simulink model "bb_pid_hg_sl"  (Simulink 7.9)
settings: Solver=FixedStepDiscrete  StartTime=0.0  StopTime=inf  FixedStep=ts  RelTol=1e-3
values from neighbouring files (symbols this model uses):
  K_theta_hg = (pi/180)*(2.1/15)    (= 0.00244346095279)    [bb_lqr_hg.m]    (also in bb_lqr_servo_hg.m; bb_lqr_test.m; bb_pid_hg.m)
  Kd = -((p1+p2)*T + 1)/K    [bb_pid_hg.m]    (also in sim_param.mat = 0)
  kd = -(p1+p2+p3)/K_b    [bb_pid_hg.m]    (also in bb_pid_rc.m)
  kff = ki/alpha    [bb_pid_hg.m]    (also in bb_pid_rc.m)
  ki = -p1*p2*p3/K_b    [bb_pid_hg.m]    (also in bb_pid_rc.m)
  Kp = p1*p2*T/K    [bb_pid_hg.m]    (also in sim_param.mat = 0)
  kp = (p1*p2 + p2*p3 + p3*p1)/K_b    [bb_pid_hg.m]    (also in bb_pid_rc.m)
  r = 60    [sim_param.mat]
  r1 = 20    [bb_lqr_hg.m]    (also in bb_lqr_servo_hg.m = 15; bb_pid_hg.m = 15; bb_pid_rc.m = 15)
  r2 = 20    [bb_lqr_hg.m]    (also in bb_lqr_servo_hg.m = 25; bb_pid_hg.m = 25; bb_pid_rc.m = 25)
  r_cyc = 4    [sim_param.mat]
  ts = 0.02    [sim_param.mat]
undefined symbols (not defined in the file or in its folder): denbd, denlpf, denpd, DiscIntNeverNeededParam, numbd, numlpf, numpd
libraries: arduino_io_lib x6, simulink x6
settings Model: Creator=hirata  LastModifiedBy=hirata
settings DebuggingCC: FcnCallInpInsideContextMsg=Use local settings
settings GRTTargetCC: CombineOutputUpdateFcns=off  GRTInterface=on

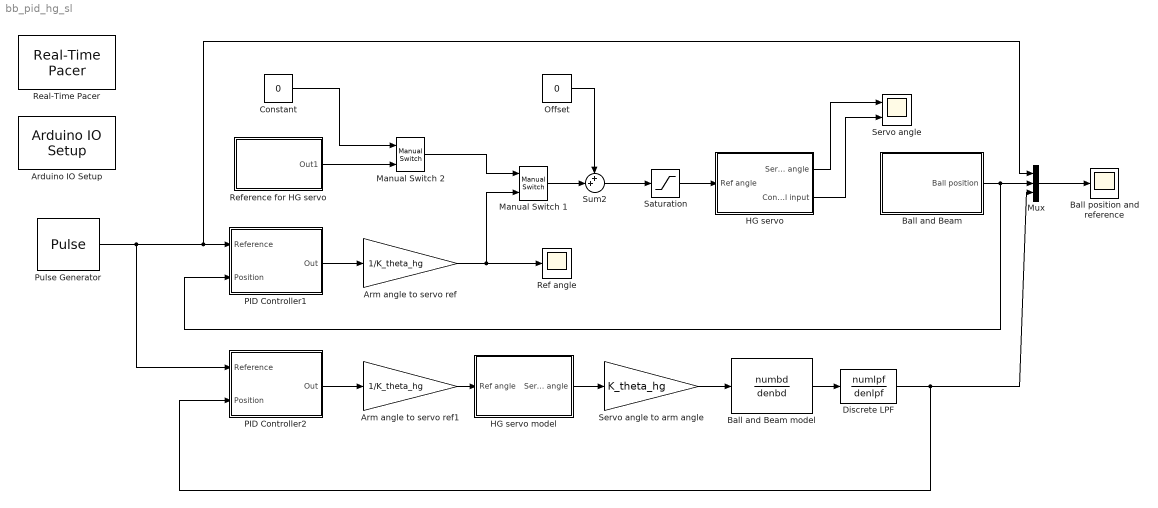
== system bb_pid_hg_sl ==
  Arduino IO Setup : arduino_io_lib/Arduino IO Setup  Priority=3  arduinoVar=Temporary arduino variable: Arduino1  workspaceVarName=a  comPort=COM3
  Arm angle to servo ref : Gain  Gain=1/K_theta_hg
  Arm angle to servo ref1 : Gain  Gain=1/K_theta_hg
  Ball and Beam : Subsystem
  Ball and Beam model : DiscreteTransferFcn  Numerator=numbd  Denominator=denbd
  Ball position and reference : Scope
      settings: TimeRange=30  YMin=-15  YMax=25
  Constant : Constant  Value=0
  Discrete LPF : DiscreteTransferFcn  Numerator=numlpf  Denominator=denlpf
  HG servo : Subsystem
  HG servo model : Subsystem
  Manual Switch 1 : simulink/Signal Routing/Manual Switch  sw=1  action=0  varsize=off
  Manual Switch 2 : simulink/Signal Routing/Manual Switch  sw=0  action=0  varsize=off
  Mux : Mux  Inputs=3
  Offset : Constant  Value=0  SampleTime=ts
  PID Controller1 : Subsystem
  PID Controller2 : Subsystem
  Pulse Generator : DiscretePulseGenerator  PulseType=Time based  Amplitude=r2-r1  Period=30  PulseWidth=50  PhaseDelay=10
  Real-Time Pacer : arduino_io_lib/Real-Time Pacer  simTimePerRealTime=1
  Ref angle : Scope
      settings: TimeRange=30  YMin=-50  YMax=50  SaveName=ScopeData5
  Reference for HG servo : Subsystem
  Saturation : Saturate  UpperLimit=45  LowerLimit=-45
  Servo angle : Scope  NumInputPorts=2
      settings: TimeRange=10  YMin=-50~-5  YMax=50~5  SaveName=ScopeData4
  Servo angle to arm angle : Gain  Gain=K_theta_hg
  Sum2 : Sum  Inputs=++|
  wires:
  Offset/1 -> Sum2/1
  Arm angle to servo ref/1 -> Manual Switch 1/2, Ref angle/1
  Sum2/1 -> Saturation/1
  Mux/1 -> Ball position and reference/1
  Manual Switch 1/1 -> Sum2/2
  Saturation/1 -> HG servo/1(Ref angle)
  Ball and Beam/1(Ball position) -> Mux/2, PID Controller1/2(Position)
  Pulse Generator/1 -> Mux/1, PID Controller1/1(Reference), PID Controller2/1(Reference)
  Ball and Beam model/1 -> Discrete LPF/1
  PID Controller1/1(Out) -> Arm angle to servo ref/1
  Discrete LPF/1 -> Mux/3, PID Controller2/2(Position)
  HG servo/1(Servo angle) -> Servo angle/1
  HG servo/2(Control input) -> Servo angle/2
  Arm angle to servo ref1/1 -> HG servo model/1(Ref angle)
  HG servo model/1(Servo angle) -> Servo angle to arm angle/1
  PID Controller2/1(Out) -> Arm angle to servo ref1/1
  Servo angle to arm angle/1 -> Ball and Beam model/1
  Manual Switch 2/1 -> Manual Switch 1/1
  Reference for HG servo/1(Out1) -> Manual Switch 2/2
  Constant/1 -> Manual Switch 2/1

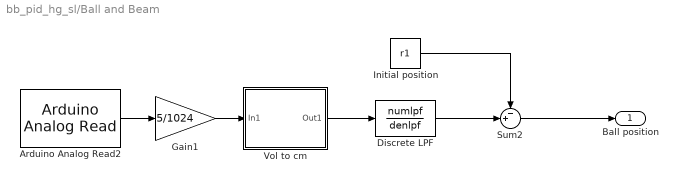
== system bb_pid_hg_sl/Ball and Beam ==
  Arduino Analog Read2 : arduino_io_lib/Arduino Analog Read  arduinoVar=Temporary arduino variable: Arduino1  arduinoPin=2  T=ts
  Discrete LPF : DiscreteTransferFcn  Numerator=numlpf  Denominator=denlpf
  Gain1 : Gain  Gain=5/1024
  Initial position : Constant  Value=r1
  Sum2 : Sum  Inputs=-+|
  Vol to cm : Subsystem
  Ball position : Outport
  wires:
  Arduino Analog Read2/1 -> Gain1/1
  Gain1/1 -> Vol to cm/1(In1)
  Vol to cm/1(Out1) -> Discrete LPF/1
  Initial position/1 -> Sum2/1
  Discrete LPF/1 -> Sum2/2
  Sum2/1 -> Ball position/1

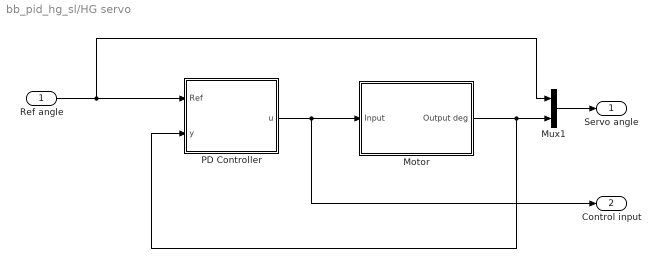
== system bb_pid_hg_sl/HG servo ==
  Ref angle : Inport
  Motor : Subsystem
  Mux1 : Mux  Inputs=2
  PD Controller : Subsystem
  Servo angle : Outport
  Control input : Outport  Port=2
  wires:
  Mux1/1 -> Servo angle/1
  Motor/1(Output deg) -> Mux1/2, PD Controller/2(y)
  Ref angle/1 -> Mux1/1, PD Controller/1(Ref)
  PD Controller/1(u) -> Motor/1(Input), Control input/1

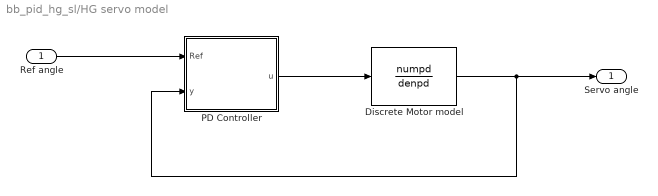
== system bb_pid_hg_sl/HG servo model ==
  Ref angle : Inport
  Discrete Motor model : DiscreteTransferFcn  Numerator=numpd  Denominator=denpd
  PD Controller : Subsystem
  Servo angle : Outport
  wires:
  Ref angle/1 -> PD Controller/1(Ref)
  PD Controller/1(u) -> Discrete Motor model/1
  Discrete Motor model/1 -> Servo angle/1, PD Controller/2(y)

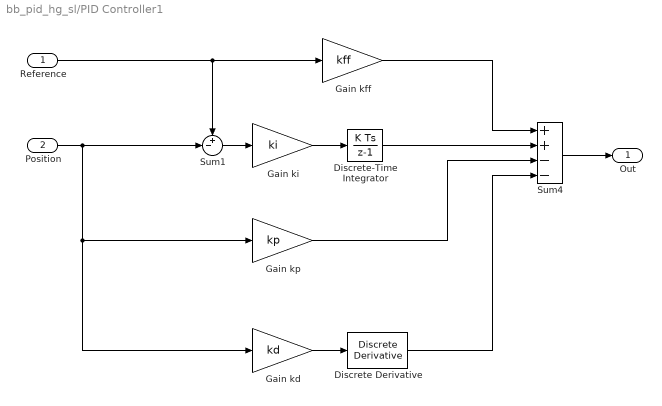
== system bb_pid_hg_sl/PID Controller1 ==
  Reference : Inport
  Position : Inport  Port=2
  Discrete Derivative : simulink/Discrete/Discrete Derivative  gainval=1.0  ICPrevScaledInput=0.0  InputProcessing=Inherited  OutMin=[]  OutMax=[]  OutDataType=fixdt(1, 16)  OutScaling=2^-10  DoSatur=off
  Discrete-Time Integrator : DiscreteIntegrator  SampleTime=ts  ICPrevOutput=DiscIntNeverNeededParam  ICPrevScaledInput=DiscIntNeverNeededParam
  Gain kd : Gain  Gain=kd
  Gain kff : Gain  Gain=kff
  Gain ki : Gain  Gain=ki
  Gain kp : Gain  Gain=kp
  Sum1 : Sum  Inputs=+-|
  Sum4 : Sum  Inputs=++--
  Out : Outport
  wires:
  Reference/1 -> Sum1/1, Gain kff/1
  Sum1/1 -> Gain ki/1
  Position/1 -> Sum1/2, Gain kp/1, Gain kd/1
  Discrete-Time Integrator/1 -> Sum4/2
  Gain ki/1 -> Discrete-Time Integrator/1
  Sum4/1 -> Out/1
  Gain kff/1 -> Sum4/1
  Gain kp/1 -> Sum4/3
  Gain kd/1 -> Discrete Derivative/1
  Discrete Derivative/1 -> Sum4/4

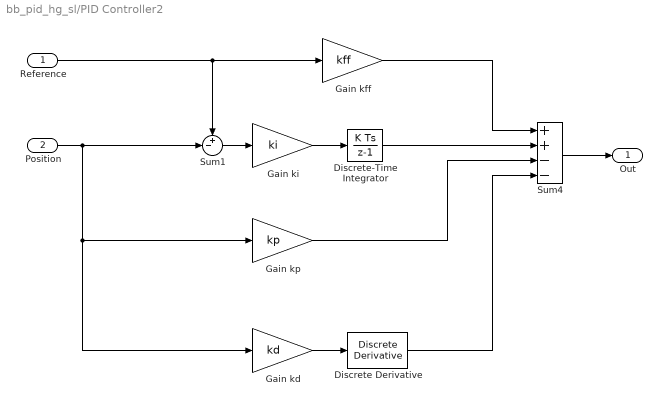
== system bb_pid_hg_sl/PID Controller2 ==
  Reference : Inport
  Position : Inport  Port=2
  Discrete Derivative : simulink/Discrete/Discrete Derivative  gainval=1.0  ICPrevScaledInput=0.0  InputProcessing=Inherited  OutMin=[]  OutMax=[]  OutDataType=fixdt(1, 16)  OutScaling=2^-10  DoSatur=off
  Discrete-Time Integrator : DiscreteIntegrator  SampleTime=ts  ICPrevOutput=DiscIntNeverNeededParam  ICPrevScaledInput=DiscIntNeverNeededParam
  Gain kd : Gain  Gain=kd
  Gain kff : Gain  Gain=kff
  Gain ki : Gain  Gain=ki
  Gain kp : Gain  Gain=kp
  Sum1 : Sum  Inputs=+-|
  Sum4 : Sum  Inputs=++--
  Out : Outport
  wires:
  Reference/1 -> Sum1/1, Gain kff/1
  Sum1/1 -> Gain ki/1
  Position/1 -> Sum1/2, Gain kp/1, Gain kd/1
  Discrete-Time Integrator/1 -> Sum4/2
  Gain ki/1 -> Discrete-Time Integrator/1
  Sum4/1 -> Out/1
  Gain kff/1 -> Sum4/1
  Gain kp/1 -> Sum4/3
  Gain kd/1 -> Discrete Derivative/1
  Discrete Derivative/1 -> Sum4/4

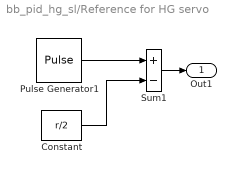
== system bb_pid_hg_sl/Reference for HG servo ==
  Constant : Constant  Value=r/2
  Pulse Generator1 : DiscretePulseGenerator  PulseType=Time based  Amplitude=r  Period=r_cyc  PulseWidth=50
  Sum1 : Sum  Inputs=+-
  Out1 : Outport
  wires:
  Pulse Generator1/1 -> Sum1/1
  Constant/1 -> Sum1/2
  Sum1/1 -> Out1/1

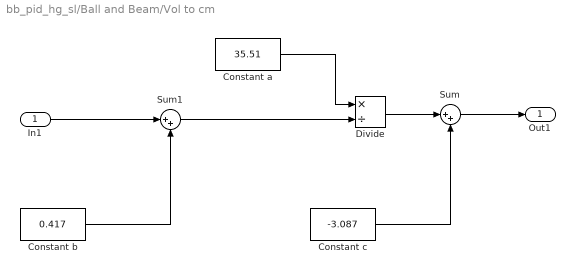
== system bb_pid_hg_sl/Ball and Beam/Vol to cm ==
  In1 : Inport
  Constant a : Constant  Value=35.51
  Constant b : Constant  Value=0.417
  Constant c : Constant  Value=-3.087
  Divide : Product  Inputs=*/
  Sum : Sum  Inputs=|++
  Sum1 : Sum  Inputs=|++
  Out1 : Outport
  wires:
  Constant a/1 -> Divide/1
  Divide/1 -> Sum/1
  Sum/1 -> Out1/1
  Constant c/1 -> Sum/2
  In1/1 -> Sum1/1
  Sum1/1 -> Divide/2
  Constant b/1 -> Sum1/2

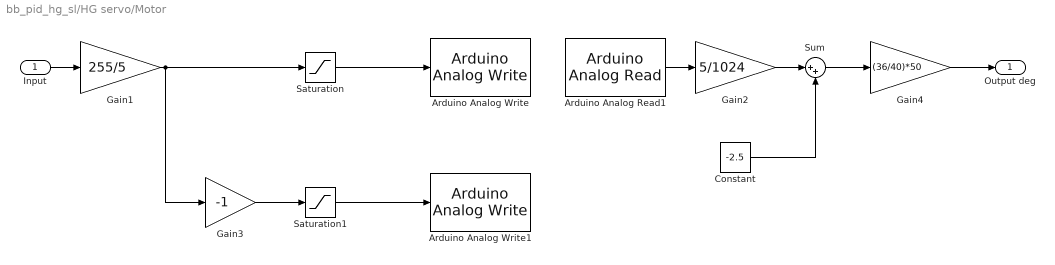
== system bb_pid_hg_sl/HG servo/Motor ==
  Input : Inport
  Arduino Analog Read1 : arduino_io_lib/Arduino Analog Read  arduinoVar=Temporary arduino variable: Arduino1  arduinoPin=0  T=ts
  Arduino Analog Write : arduino_io_lib/Arduino Analog Write  arduinoVar=Temporary arduino variable: Arduino1  arduinoPin=3  T=ts
  Arduino Analog Write1 : arduino_io_lib/Arduino Analog Write  arduinoVar=Temporary arduino variable: Arduino1  arduinoPin=5  T=ts
  Constant : Constant  Value=-2.5
  Gain1 : Gain  Gain=255/5
  Gain2 : Gain  Gain=5/1024
  Gain3 : Gain  Gain=-1
  Gain4 : Gain  Gain=(36/40)*50
  Saturation : Saturate  UpperLimit=255  LowerLimit=0
  Saturation1 : Saturate  UpperLimit=255  LowerLimit=0
  Sum : Sum  Inputs=|++
  Output deg : Outport
  wires:
  Gain3/1 -> Saturation1/1
  Constant/1 -> Sum/2
  Sum/1 -> Gain4/1
  Gain2/1 -> Sum/1
  Gain4/1 -> Output deg/1
  Saturation1/1 -> Arduino Analog Write1/1
  Gain1/1 -> Saturation/1, Gain3/1
  Saturation/1 -> Arduino Analog Write/1
  Arduino Analog Read1/1 -> Gain2/1
  Input/1 -> Gain1/1

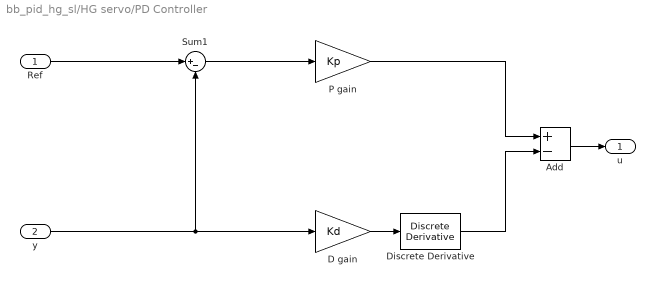
== system bb_pid_hg_sl/HG servo/PD Controller ==
  Ref : Inport
  y : Inport  Port=2
  Add : Sum  Inputs=+-
  D gain : Gain  Gain=Kd
  Discrete Derivative : simulink/Discrete/Discrete Derivative  gainval=1.0  ICPrevScaledInput=0.0  InputProcessing=Inherited  OutMin=[]  OutMax=[]  OutDataType=fixdt(1, 16)  OutScaling=2^-10  DoSatur=off
  P gain : Gain  Gain=Kp
  Sum1 : Sum  Inputs=|+-
  u : Outport
  wires:
  D gain/1 -> Discrete Derivative/1
  Discrete Derivative/1 -> Add/2
  Add/1 -> u/1
  Ref/1 -> Sum1/1
  P gain/1 -> Add/1
  y/1 -> D gain/1, Sum1/2
  Sum1/1 -> P gain/1

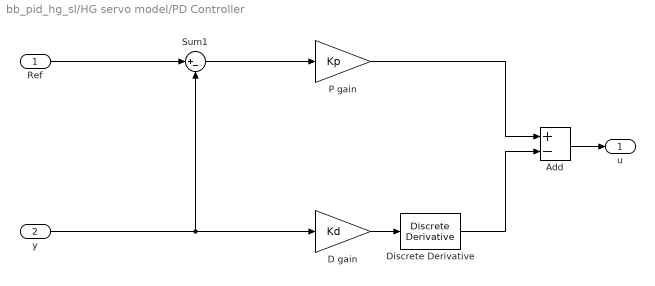
== system bb_pid_hg_sl/HG servo model/PD Controller ==
  Ref : Inport
  y : Inport  Port=2
  Add : Sum  Inputs=+-
  D gain : Gain  Gain=Kd
  Discrete Derivative : simulink/Discrete/Discrete Derivative  gainval=1.0  ICPrevScaledInput=0.0  InputProcessing=Inherited  OutMin=[]  OutMax=[]  OutDataType=fixdt(1, 16)  OutScaling=2^-10  DoSatur=off
  P gain : Gain  Gain=Kp
  Sum1 : Sum  Inputs=|+-
  u : Outport
  wires:
  Sum1/1 -> P gain/1
  y/1 -> Sum1/2, D gain/1
  P gain/1 -> Add/1
  Ref/1 -> Sum1/1
  Add/1 -> u/1
  Discrete Derivative/1 -> Add/2
  D gain/1 -> Discrete Derivative/1
